simulink model "ejemplo_2_leer_odometria"  (R2026a)
settings: Solver=VariableStepAuto  StopTime=inf
libraries: ros2lib x1
settings Model: Creator=samuel  LastModifiedBy=samuel

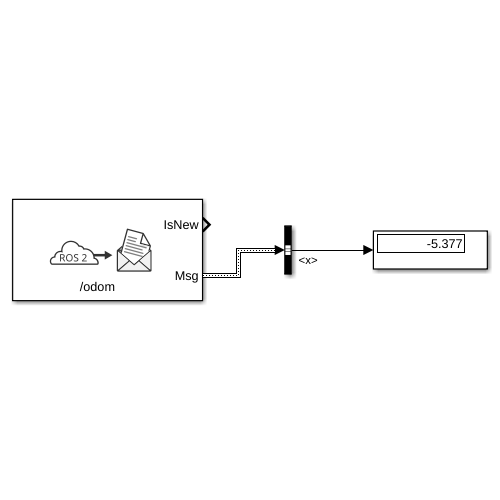
[thumbnail: Simulink's stored preview of the top-level diagram]
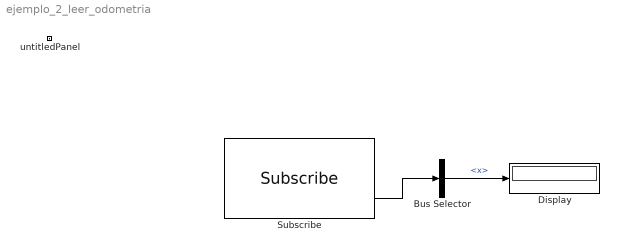
== system ejemplo_2_leer_odometria ==
  Bus Selector : BusSelector  OutputSignals=pose.pose.position.x
  Display : Display
  Subscribe : ros2lib/Subscribe  topicSource=Specify your own  topic=/odom  messageType=nav_msgs/Odometry  sampleTime=-1  QOSHistory=Keep last  QOSDepth=10  QOSReliability=Reliable  QOSDurability=Volatile  QOSDeadline=Inf  QOSLifespan=Inf  QOSLiveliness=Automatic  QOSLeaseDuration=Inf  QOSAvoidROSNamespaceConventions=off
  untitledPanel : Subsystem  Tag=HiddenForWebPanel  IsWebBlockPanel=on
  wires:
  Subscribe/2 -> Bus Selector/1
  Bus Selector/1 -> Display/1  "<x>"

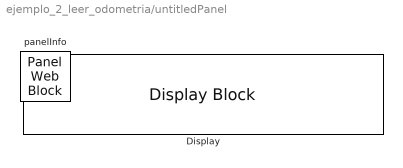
== system ejemplo_2_leer_odometria/untitledPanel ==
  Display : DisplayBlock  Tag=HiddenForWebPanel  PanelInfo="{\"height\":80,\"left\":18,\"panelId\":\"panelId-83ea5b45-7469-4072-9039-4239fb6e5d39\",\"top\":18,\"type\":\"panelChild\",\"version\":\"2019b\",\"width\":360,\"zIndex\":1500002}"  LabelPosition=Hide  Transparency=1  GridColor=[0.502, 0.502, 0.502]
  panelInfo : PanelWebBlock  Tag=HiddenForWebPanel  PanelInfo="{\"compacted\":false,\"height\":120,\"isActiveTab\":true,\"left\":486,\"name\":\"Panel\",\"panelId\":\"panelId-83ea5b45-7469-4072-9039-4239fb6e5d39\",\"popoutData\":{\"height\":0,\"left\":0,\"maximized\":false,\"top\":0,\"width\":0},\"popoutMode\":\"componentHidden\",\"tabIndex\":0,\"tabbedSetId\":\"tabbedSet6232451427\",\"top\":245,\"type\":\"panel\",\"version\":\"2019b\",\"visible\":true,\"width\":400,\"zIndex\":1500002}"
